simulink model "SWC_FDC_type"  (R2021b)
settings: Solver=FixedStepDiscrete  StartTime=0.0  StopTime=10.0  FixedStep=0.001  RelTol=1e-3
values from neighbouring files (symbols this model uses):
  DID_VCUKey = uint16(0x0202)    [vcu_local_hdr.m]
  DID_XWD = uint16(513)    [vcu_local_hdr.m]
  DIDLen_DKCKey = uint16(8)    [vcu_local_hdr.m]
  DIDLen_DynoMode = uint16(1)    [vcu_local_hdr.m]
  DIDLen_LFLowPresThre = uint16(1)    [vcu_local_hdr.m]
  DIDLen_LFSensorID = uint16(4)    [vcu_local_hdr.m]
  DIDLen_LRLowPresThre = uint16(1)    [vcu_local_hdr.m]
  DIDLen_LRSensorID = uint16(4)    [vcu_local_hdr.m]
  DIDLen_RFLowPresThre = uint16(1)    [vcu_local_hdr.m]
  DIDLen_RFSensorID = uint16(4)    [vcu_local_hdr.m]
  DIDLen_RRLowPresThre = uint16(1)    [vcu_local_hdr.m]
  DIDLen_RRSensorID = uint16(4)    [vcu_local_hdr.m]
  DIDLen_SensorMode = uint16(1)    [vcu_local_hdr.m]
  DIDLen_TPMSLearnSta = uint16(1)    [vcu_local_hdr.m]
  DIDLen_WhlPres = uint16(4)    [vcu_local_hdr.m]
  DIDLen_WhlSensorBattSta = uint16(1)    [vcu_local_hdr.m]
  DIDLen_WhlTmp = uint16(4)    [vcu_local_hdr.m]
  DIDLen_XWDMode = uint16(1)    [vcu_local_hdr.m]
  DIDNum_DKCKey = uint16(0x0202)    [vcu_local_hdr.m]
  DIDNum_DynoMode = uint16(0x0203)    [vcu_local_hdr.m]
  DIDNum_LFLowPresThre = uint16(0x0B08)    [vcu_local_hdr.m]
  DIDNum_LFSensorID = uint16(0x0B01)    [vcu_local_hdr.m]
  DIDNum_LRLowPresThre = uint16(0x0B0A)    [vcu_local_hdr.m]
  DIDNum_LRSensorID = uint16(0x0B03)    [vcu_local_hdr.m]
  DIDNum_RFLowPresThre = uint16(0x0B09)    [vcu_local_hdr.m]
  DIDNum_RFSensorID = uint16(0x0B02)    [vcu_local_hdr.m]
  DIDNum_RRLowPresThre = uint16(0x0B0B)    [vcu_local_hdr.m]
  DIDNum_RRSensorID = uint16(0x0B04)    [vcu_local_hdr.m]
  DIDNum_SensorMode = uint16(0x0B0C)    [vcu_local_hdr.m]
  DIDNum_TPMSLearnSta = uint16(0x0B0D)    [vcu_local_hdr.m]
  DIDNum_WhlPres = uint16(0x0B05)    [vcu_local_hdr.m]
  DIDNum_WhlSensorBattSta = uint16(0x0B07)    [vcu_local_hdr.m]
  DIDNum_WhlTmp = uint16(0x0B06)    [vcu_local_hdr.m]
  DIDNum_XWDMode = uint16(0x0201)    [vcu_local_hdr.m]
  DIDVCUKeyLength = uint16(8)    [vcu_local_hdr.m]
  ENUM_DRIVETRAIN_AWD = uint8(  2  )    [vcu_local_hdr.m]
  ENUM_DRIVETRAIN_FWD = uint8(  1  )    [vcu_local_hdr.m]
  ENUM_DRIVETRAIN_RWD = uint8(  0  )    [vcu_local_hdr.m]
  ENUM_TPMSLearnStatus_LEARNED = uint8(  1  )    [vcu_local_hdr.m]
  ENUM_TPMSLearnStatus_LEARNFAIL = uint8(  2  )    [vcu_local_hdr.m]
  ENUM_TPMSLearnStatus_NOTLEARN = uint8(  0  )    [vcu_local_hdr.m]
  ENUM_TPMSSTA_FAT = uint8(  8  )    [vcu_local_hdr.m]
  ENUM_TPMSSTA_LOWBATTERY = uint8(  2  )    [vcu_local_hdr.m]
  FALSE = boolean( 0 )    [vcu_local_hdr.m]
  ONE_INT = uint8(1)    [vcu_local_hdr.m]
  P_boolean = 0.0    [APPTypes.sldd]
  TRUE = boolean( 1 )    [vcu_local_hdr.m]
  ZERO_FLOAT = single(0)    [vcu_local_hdr.m]
  ZERO_INT = uint8(0)    [vcu_local_hdr.m]
undefined symbols (not defined in the file or in its folder): f32_ApsOutVehSpdSig, KHAL_DKCDecryptEnable_flg_ovrdflg, KHAL_DKCDecryptEnable_flg_ovrdval, KHAL_RandomNumberY1_enum, KHAL_RandomNumberY2_enum, KHAL_RandomNumberY_ovrdflg, KHAL_TPMSRESBUTT_flg_ovrdflg, KHAL_TPMSRESBUTT_flg_ovrdval, R_DIDWriteCDD_CSOP_DIDSet_DKCKey, R_DIDWriteCDD_CSOP_DIDSet_DynoMode, R_DIDWriteCDD_CSOP_DIDSet_LFLowPresThre, R_DIDWriteCDD_CSOP_DIDSet_LFSensorID, R_DIDWriteCDD_CSOP_DIDSet_LRLowPresThre, R_DIDWriteCDD_CSOP_DIDSet_LRSensorID, R_DIDWriteCDD_CSOP_DIDSet_RFLowPresThre, R_DIDWriteCDD_CSOP_DIDSet_RFSensorID, R_DIDWriteCDD_CSOP_DIDSet_RRLowPresThre, R_DIDWriteCDD_CSOP_DIDSet_RRSensorID, R_DIDWriteCDD_CSOP_DIDSet_SensorMode, R_DIDWriteCDD_CSOP_DIDSet_TPMSLearnSta, R_DIDWriteCDD_CSOP_DIDSet_WhlPres, R_DIDWriteCDD_CSOP_DIDSet_WhlSensorBattSta, R_DIDWriteCDD_CSOP_DIDSet_WhlTmp, R_DIDWriteCDD_CSOP_DIDSet_XWDMode, R_E2E_CAN3_VCU1_CSOP_Write_CAN3_VCU1, R_E2E_CAN4_VCU1_CSOP_Write_CAN4_VCU1, R_FDCCDD_Inner_CSOP_FDC_AppCallSleep, R_HALIN_IMU_CSOP_IMUSetSta, R_HALINCDD_CSOP_PAS_Handler, R_HALINCDD_CSOP_UDS_Main, R_HALOUT_APS_CSOP_ApsOutput, R_HALOUTCDD_CSOP_AppNmStateReq, R_HALOUTCDD_CSOP_IVIReset, R_HALOUTCDD_CSOP_SetAcoreRebootCmdACK, R_HALOUTCDD_CSOP_SetSysPwrStat, R_HALOUTCDD_CSOP_SleepRequest, R_NVMReadCDD_Inner_NVM_ReadOperation, R_NVMWriteCDD_Inner_NVM_WriteOperation, R_UDSCDD_CSOP_DdmRestartOperationCycle, R_WDGCDD_CSOP_Call_Watchdog, R_WDGCDD_CSOP_Call_WDG_AppEnd, R_WDGCDD_CSOP_Call_WDG_AppStart, u16_DIDLen_DKCKey, u16_DIDLen_DynoMode, u16_DIDLen_LFLowPresThre, u16_DIDLen_LFSensorID, u16_DIDLen_LRLowPresThre, u16_DIDLen_LRSensorID, u16_DIDLen_RFLowPresThre, u16_DIDLen_RFSensorID, u16_DIDLen_RRLowPresThre, u16_DIDLen_RRSensorID, u16_DIDLen_SensorMode, u16_DIDLen_TPMSLearnSta, u16_DIDLen_WhlPres, u16_DIDLen_WhlSensorBattSta, u16_DIDLen_WhlTmp, u16_DIDLen_XWDMode, u16_DIDNum_DKCKey, u16_DIDNum_DynoMode ... (+42)
libraries: simulink x215, FVT_lib x137, hcu_lib x12, hdlsllib x9, app x1, halin x1, halout x1, inp x1, outp x1
(part 6 of 11)

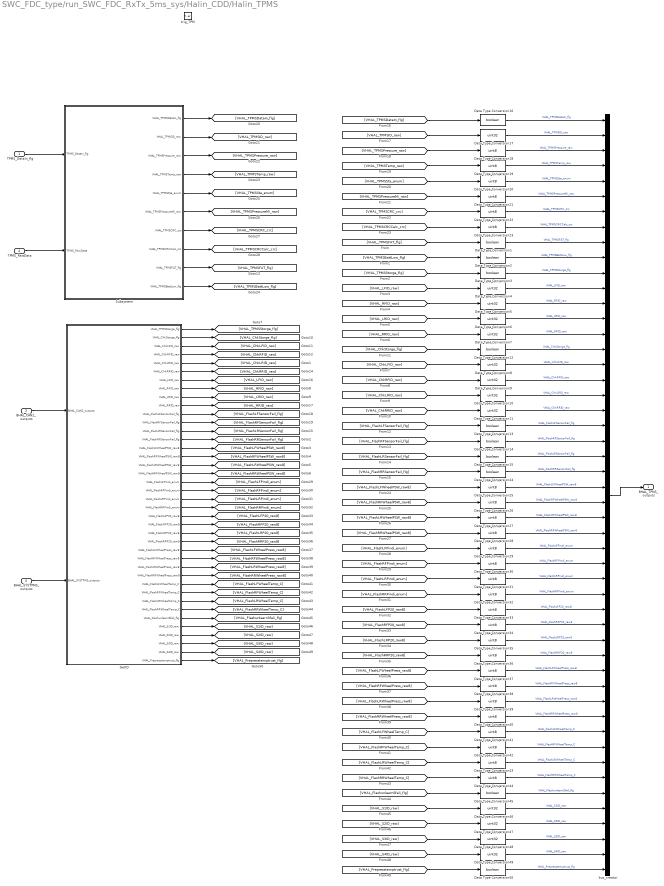
== system SWC_FDC_type/run_SWC_FDC_RxTx_5ms_sys/Halin_CDD/Halin_TPMS ==
  TPMS_DataIn_flg : Inport
  TPMS_RawData : Inport  Port=2
  BHAL_CAN2_outputs : Inport  Port=3
  BHAL_SYSTPMS_outputs : Inport  Port=4
  trig_TPM : TriggerPort  TriggerType=function-call  VariantControl=(inherit)
  Data Type Conversion{1..3,12..16,24,45,50} (11 alike) : DataTypeConversion  OutDataTypeStr=boolean
  Data Type Conversion{4..11,17,46..49} (13 alike) : DataTypeConversion  OutDataTypeStr=uint32
  Data Type Conversion{18..23,25..44} (26 alike) : DataTypeConversion  OutDataTypeStr=uint8
  GetID : Subsystem
  Subsystem : Subsystem
  bus_creator : BusCreator  Inputs=50  OutDataTypeStr=Bus: BHAL_TPMS_outputs  NonVirtualBus=on
  BHAL_TPMS_outputs : Outport
  wires:
  Subsystem/8(VHAL_TPMSCRCCalc_crc) -> [VHAL_TPMSCRCCalc_crc]
  Subsystem/7(VHAL_TPMSCRC_crc) -> [VHAL_TPMSCRC_crc]
  Subsystem/1(VHAL_TPMSDataIn_flg) -> [VHAL_TPMSDataIn_flg]
  Subsystem/9(VHAL_TPMSFAT_flg) -> [VHAL_TPMSFAT_flg]
  Subsystem/2(VHAL_TPMSID_raw) -> [VHAL_TPMSID_raw]
  Subsystem/10(VHAL_TPMSBattLow_flg) -> [VHAL_TPMSBattLow_flg]
  Subsystem/4(VHAL_TPMSTemp_raw) -> [VHAL_TPMSTemp_raw]
  Subsystem/5(VHAL_TPMSSta_enum) -> [VHAL_TPMSSta_enum]
  Subsystem/3(VHAL_TPMSPressure_raw) -> [VHAL_TPMSPressure_raw]
  Subsystem/6(VHAL_TPMSPressureMi_raw) -> [VHAL_TPMSPressureMi_raw]
  TPMS_DataIn_flg/1 -> Subsystem/1(TPMS_DataIn_flg)
  TPMS_RawData/1 -> Subsystem/2(TPMS_RawData)
  Data Type Conversion29/1 -> bus_creator/29  "VHAL_FlashLFPindi_enum"
  GetID/20(VHAL_FlashRFPindi_enum) -> [VHAL_FlashRFPindi_enum]
  GetID/32(VHAL_FlashRFWheelTemp_C) -> [VHAL_FlashRFWheelTemp_C]
  Data Type Conversion2/1 -> bus_creator/10  "VHAL_TPMSBattLow_flg"
  BHAL_CAN2_outputs/1 -> GetID/1(BHAL_CAN2_outputs)
  [VHAL_TPMSBattLow_flg] -> Data Type Conversion2/1
  [VHAL_FlashLRPindi_enum] -> Data Type Conversion31/1
  [VHAL_FlashunlearnSfali_flg] -> Data Type Conversion45/1
  [VHAL_FlashLFPindi_enum] -> Data Type Conversion29/1
  Data Type Conversion28/1 -> bus_creator/28  "VHAL_FlashRRWheelPSW_raw8"
  [VHAL_FlashLFP20_raw8] -> Data Type Conversion33/1
  [VHAL_RRID_raw] -> Data Type Conversion7/1
  Data Type Conversion42/1 -> bus_creator/42  "VHAL_FlashRFWheelTemp_C"
  Data Type Conversion27/1 -> bus_creator/27  "VHAL_FlashLRWheelPSW_raw8"
  [VHAL_FlashLFWheelTemp_C] -> Data Type Conversion41/1
  Data Type Conversion26/1 -> bus_creator/26  "VHAL_FlashRFWheelPSW_raw8"
  [VHAL_FlashRRP20_raw8] -> Data Type Conversion36/1
  GetID/16(VHAL_FlashRFWheelPSW_raw8) -> [VHAL_FlashRFWheelPSW_raw8]
  [VHAL_RFID_raw] -> Data Type Conversion5/1
  Data Type Conversion33/1 -> bus_creator/33  "VHAL_FlashLFP20_raw8"
  Data Type Conversion24/1 -> bus_creator/24  "VHAL_FlashRRSensorFail_flg"
  Data Type Conversion44/1 -> bus_creator/44  "VHAL_FlashRRWheelTemp_C"
  Data Type Conversion34/1 -> bus_creator/34  "VHAL_FlashRFP20_raw8"
  Data Type Conversion45/1 -> bus_creator/45  "VHAL_FlashunlearnSfali_flg"
  GetID/9(VHAL_LRID_raw) -> [VHAL_LRID_raw]
  Data Type Conversion41/1 -> bus_creator/41  "VHAL_FlashLFWheelTemp_C"
  GetID/15(VHAL_FlashLFWheelPSW_raw8) -> [VHAL_FlashLFWheelPSW_raw8]
  Data Type Conversion15/1 -> bus_creator/23  "VHAL_FlashLRSensorFail_flg"
  [VHAL_FlashLRWheelPress_raw8] -> Data Type Conversion39/1
  Data Type Conversion14/1 -> bus_creator/22  "VHAL_FlashRFSensorFail_flg"
  GetID/34(VHAL_FlashRRWheelTemp_C) -> [VHAL_FlashRRWheelTemp_C]
  Data Type Conversion13/1 -> bus_creator/21  "VHAL_FlashLFSensorFail_flg"
  Data Type Conversion32/1 -> bus_creator/32  "VHAL_FlashRRPindi_enum"
  Data Type Conversion31/1 -> bus_creator/31  "VHAL_FlashLRPindi_enum"
  Data Type Conversion16/1 -> bus_creator/1  "VHAL_TPMSDataIn_flg"
  GetID/22(VHAL_FlashRRPindi_enum) -> [VHAL_FlashRRPindi_enum]
  [VHAL_FlashRFSensorFail_flg] -> Data Type Conversion14/1
  GetID/18(VHAL_FlashRRWheelPSW_raw8) -> [VHAL_FlashRRWheelPSW_raw8]
  Data Type Conversion43/1 -> bus_creator/43  "VHAL_FlashLRWheelTemp_C"
  Data Type Conversion22/1 -> bus_creator/7  "VHAL_TPMSCRC_crc"
  Data Type Conversion40/1 -> bus_creator/40  "VHAL_FlashRRWheelPress_raw8"
  Data Type Conversion39/1 -> bus_creator/39  "VHAL_FlashLRWheelPress_raw8"
  [VHAL_FlashRRPindi_enum] -> Data Type Conversion32/1
  Data Type Conversion38/1 -> bus_creator/38  "VHAL_FlashRFWheelPress_raw8"
  [VHAL_FlashLRP20_raw8] -> Data Type Conversion35/1
  Data Type Conversion35/1 -> bus_creator/35  "VHAL_FlashLRP20_raw8"
  GetID/14(VHAL_FlashRRSensorFail_flg) -> [VHAL_FlashRRSensorFail_flg]
  Data Type Conversion37/1 -> bus_creator/37  "VHAL_FlashLFWheelPress_raw8"
  Data Type Conversion36/1 -> bus_creator/36  "VHAL_FlashRRP20_raw8"
  [VHAL_FlashRRWheelTemp_C] -> Data Type Conversion44/1
  [VHAL_FlashLFWheelPress_raw8] -> Data Type Conversion37/1
  GetID/33(VHAL_FlashLRWheelTemp_C) -> [VHAL_FlashLRWheelTemp_C]
  GetID/26(VHAL_FlashRRP20_raw8) -> [VHAL_FlashRRP20_raw8]
  [VHAL_TPMSFAT_flg] -> Data Type Conversion1/1
  [VHAL_TPMSSta_enum] -> Data Type Conversion20/1
  GetID/25(VHAL_FlashLRP20_raw8) -> [VHAL_FlashLRP20_raw8]
  [VHAL_FlashRRWheelPress_raw8] -> Data Type Conversion40/1
  [VHAL_FlashRFP20_raw8] -> Data Type Conversion34/1
  [VHAL_LFID_raw] -> Data Type Conversion4/1
  [VHAL_FlashRFWheelPSW_raw8] -> Data Type Conversion26/1
  [VHAL_FlashRFWheelTemp_C] -> Data Type Conversion42/1
  [VHAL_FlashLRWheelTemp_C] -> Data Type Conversion43/1
  [VHAL_TPMSCRCCalc_crc] -> Data Type Conversion23/1
  GetID/31(VHAL_FlashLFWheelTemp_C) -> [VHAL_FlashLFWheelTemp_C]
  [VHAL_FlashRRSensorFail_flg] -> Data Type Conversion24/1
  [VHAL_FlashLFSensorFail_flg] -> Data Type Conversion13/1
  GetID/30(VHAL_FlashRRWheelPress_raw8) -> [VHAL_FlashRRWheelPress_raw8]
  Data Type Conversion3/1 -> bus_creator/11  "VHAL_TPMSStorge_flg"
  GetID/29(VHAL_FlashLRWheelPress_raw8) -> [VHAL_FlashLRWheelPress_raw8]
  GetID/21(VHAL_FlashLRPindi_enum) -> [VHAL_FlashLRPindi_enum]
  GetID/1(VHAL_TPMSStorge_flg) -> [VHAL_TPMSStorge_flg]
  [VHAL_FlashRFPindi_enum] -> Data Type Conversion30/1
  GetID/19(VHAL_FlashLFPindi_enum) -> [VHAL_FlashLFPindi_enum]
  GetID/23(VHAL_FlashLFP20_raw8) -> [VHAL_FlashLFP20_raw8]
  Data Type Conversion6/1 -> bus_creator/14  "VHAL_LRID_raw"
  GetID/6(VHAL_ChkRRID_raw) -> [VHAL_ChkRRID_raw]
  [VHAL_TPMSDataIn_flg] -> Data Type Conversion16/1
  GetID/17(VHAL_FlashLRWheelPSW_raw8) -> [VHAL_FlashLRWheelPSW_raw8]
  [VHAL_FlashRFWheelPress_raw8] -> Data Type Conversion38/1
  Data Type Conversion1/1 -> bus_creator/9  "VHAL_TPMSFAT_flg"
  GetID/3(VHAL_ChkLFID_raw) -> [VHAL_ChkLFID_raw]
  GetID/35(VHAL_FlashunlearnSfali_flg) -> [VHAL_FlashunlearnSfali_flg]
  [VHAL_FlashLFWheelPSW_raw8] -> Data Type Conversion25/1
  GetID/8(VHAL_RFID_raw) -> [VHAL_RFID_raw]
  GetID/10(VHAL_RRID_raw) -> [VHAL_RRID_raw]
  Data Type Conversion12/1 -> bus_creator/16  "VHAL_ChkStorge_flg"
  [VHAL_FlashLRWheelPSW_raw8] -> Data Type Conversion27/1
  GetID/7(VHAL_LFID_raw) -> [VHAL_LFID_raw]
  Data Type Conversion18/1 -> bus_creator/3  "VHAL_TPMSPressure_raw"
  Data Type Conversion9/1 -> bus_creator/18  "VHAL_ChkRFID_raw"
  Data Type Conversion10/1 -> bus_creator/19  "VHAL_ChkLRID_raw"
  GetID/11(VHAL_FlashLFSensorFail_flg) -> [VHAL_FlashLFSensorFail_flg]
  GetID/27(VHAL_FlashLFWheelPress_raw8) -> [VHAL_FlashLFWheelPress_raw8]
  Data Type Conversion11/1 -> bus_creator/20  "VHAL_ChkRRID_raw"
  Data Type Conversion7/1 -> bus_creator/15  "VHAL_RRID_raw"
  GetID/4(VHAL_ChkRFID_raw) -> [VHAL_ChkRFID_raw]
  [VHAL_TPMSID_raw] -> Data Type Conversion17/1
  [VHAL_ChkStorge_flg] -> Data Type Conversion12/1
  GetID/28(VHAL_FlashRFWheelPress_raw8) -> [VHAL_FlashRFWheelPress_raw8]
  Data Type Conversion8/1 -> bus_creator/17  "VHAL_ChkLFID_raw"
  [VHAL_ChkRRID_raw] -> Data Type Conversion11/1
  Data Type Conversion4/1 -> bus_creator/12  "VHAL_LFID_raw"
  [VHAL_ChkLRID_raw] -> Data Type Conversion10/1
  [VHAL_ChkLFID_raw] -> Data Type Conversion8/1
  [VHAL_ChkRFID_raw] -> Data Type Conversion9/1
  Data Type Conversion5/1 -> bus_creator/13  "VHAL_RFID_raw"
  [VHAL_LRID_raw] -> Data Type Conversion6/1
  [VHAL_TPMSStorge_flg] -> Data Type Conversion3/1
  GetID/2(VHAL_ChkStorge_flg) -> [VHAL_ChkStorge_flg]
  [VHAL_TPMSCRC_crc] -> Data Type Conversion22/1
  Data Type Conversion19/1 -> bus_creator/4  "VHAL_TPMSTemp_raw"
  BHAL_SYSTPMS_outputs/1 -> GetID/2(BHAL_SYSTPMS_outputs)
  [VHAL_FlashLRSensorFail_flg] -> Data Type Conversion15/1
  Data Type Conversion17/1 -> bus_creator/2  "VHAL_TPMSID_raw"
  Data Type Conversion23/1 -> bus_creator/8  "VHAL_TPMSCRCCalc_crc"
  Data Type Conversion30/1 -> bus_creator/30  "VHAL_FlashRFPindi_enum"
  Data Type Conversion21/1 -> bus_creator/6  "VHAL_TPMSPressureMi_raw"
  GetID/5(VHAL_ChkLRID_raw) -> [VHAL_ChkLRID_raw]
  [VHAL_TPMSTemp_raw] -> Data Type Conversion19/1
  GetID/13(VHAL_FlashLRSensorFail_flg) -> [VHAL_FlashLRSensorFail_flg]
  [VHAL_TPMSPressure_raw] -> Data Type Conversion18/1
  GetID/24(VHAL_FlashRFP20_raw8) -> [VHAL_FlashRFP20_raw8]
  bus_creator/1 -> BHAL_TPMS_outputs/1
  Data Type Conversion20/1 -> bus_creator/5  "VHAL_TPMSSta_enum"
  Data Type Conversion25/1 -> bus_creator/25  "VHAL_FlashLFWheelPSW_raw8"
  [VHAL_TPMSPressureMi_raw] -> Data Type Conversion21/1
  GetID/12(VHAL_FlashRFSensorFail_flg) -> [VHAL_FlashRFSensorFail_flg]
  [VHAL_FlashRRWheelPSW_raw8] -> Data Type Conversion28/1
  GetID/36(VHAL_S1ID_raw) -> [VHAL_S1ID_raw]
  GetID/37(VHAL_S2ID_raw) -> [VHAL_S2ID_raw]
  GetID/38(VHAL_S3ID_raw) -> [VHAL_S3ID_raw]
  GetID/39(VHAL_S4ID_raw) -> [VHAL_S4ID_raw]
  Data Type Conversion46/1 -> bus_creator/46  "VHAL_S1ID_raw"
  Data Type Conversion49/1 -> bus_creator/49  "VHAL_S4ID_raw"
  Data Type Conversion48/1 -> bus_creator/48  "VHAL_S3ID_raw"
  Data Type Conversion47/1 -> bus_creator/47  "VHAL_S2ID_raw"
  [VHAL_S1ID_raw] -> Data Type Conversion46/1
  [VHAL_S2ID_raw] -> Data Type Conversion47/1
  [VHAL_S3ID_raw] -> Data Type Conversion48/1
  [VHAL_S4ID_raw] -> Data Type Conversion49/1
  GetID/40(VHAL_Prepresstemptrust_flg) -> [VHAL_Prepresstemptrust_flg]
  [VHAL_Prepresstemptrust_flg] -> Data Type Conversion50/1
  Data Type Conversion50/1 -> bus_creator/50  "VHAL_Prepresstemptrust_flg"

== system SWC_FDC_type/run_SWC_FDC_RxTx_5ms_sys/Halin_CDD/Subsystem ==
  VHAL_ClearDTCcmd_flg : Inport
  Bus Creator : BusCreator  Inputs=1
  Data Type Conversion : DataTypeConversion  OutDataTypeStr=boolean
  BHAL_DDM_outputs : Outport  OutDataTypeStr=Bus: BHAL_DDM_outputs
  wires:
  VHAL_ClearDTCcmd_flg/1 -> Data Type Conversion/1
  Bus Creator/1 -> BHAL_DDM_outputs/1
  Data Type Conversion/1 -> Bus Creator/1  "VHAL_ClearDTCcmd_flg"

== system SWC_FDC_type/run_SWC_FDC_RxTx_5ms_sys/OUTP_AFTER/APM ==
  BOUTP_outputs : Inport  OutDataTypeStr=Bus: BOUTP_outputs
  Bus Selector : BusSelector  OutputSignals=VOUTP_VehSpeed_kph,VOUTP_ShiftGearPosn_enum,VOUTP_FSOffSw_enum,VOUTP_VehSpeedTimeOut_flg,VOUTP_FSOffSwTimeOut_flg,VOUTP_ChrgPlugSta_enum
  Data Type Conversion : DataTypeConversion  OutDataTypeStr=single
  Data Type Conversion{1..5} (5 alike) : DataTypeConversion  OutDataTypeStr=uint8
  ApsOut_GearPosnSig : Outport
  ApsOut_SendChrgPlugStaSig : Outport  Port=2
  ApsOut_SetFrSensorOnCmd : Outport  Port=3
  ApsOut_SetFrSensorSwTOCmd : Outport  Port=4
  ApsOut_SetVehSpdTOCmd : Outport  Port=5
  ApsOut_VehSpdSig : Outport  Port=6
  wires:
  BOUTP_outputs/1 -> [BOUTP_outputs]
  [BOUTP_outputs] -> Bus Selector/1
  Bus Selector/1 -> Data Type Conversion/1  "<VOUTP_VehSpeed_kph>"
  Bus Selector/2 -> Data Type Conversion1/1  "<VOUTP_ShiftGearPosn_enum>"
  Bus Selector/3 -> Data Type Conversion2/1  "<VOUTP_FSOffSw_enum>"
  Bus Selector/4 -> Data Type Conversion3/1  "<VOUTP_VehSpeedTimeOut_flg>"
  Bus Selector/5 -> Data Type Conversion4/1  "<VOUTP_FSOffSwTimeOut_flg>"
  Data Type Conversion1/1 -> ApsOut_GearPosnSig/1
  Data Type Conversion2/1 -> ApsOut_SetFrSensorOnCmd/1
  Data Type Conversion4/1 -> ApsOut_SetFrSensorSwTOCmd/1
  Data Type Conversion5/1 -> ApsOut_SendChrgPlugStaSig/1
  Bus Selector/6 -> Data Type Conversion5/1  "<VOUTP_ChrgPlugSta_enum>"
  Data Type Conversion/1 -> ApsOut_VehSpdSig/1
  Data Type Conversion3/1 -> ApsOut_SetVehSpdTOCmd/1

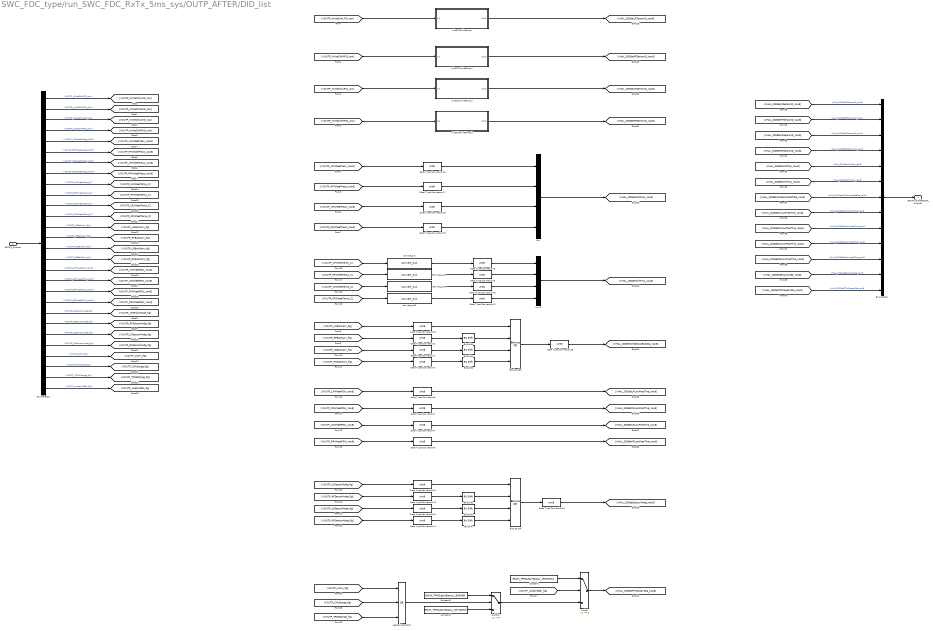
== system SWC_FDC_type/run_SWC_FDC_RxTx_5ms_sys/OUTP_AFTER/DID_list ==
  BOUTP_outputs : Inport
  Bit Shift : hdlsllib/Logic and Bit Operations/Bit Shift  mode=Shift Left Logical  N=3
  Bit Shift1 : hdlsllib/Logic and Bit Operations/Bit Shift  mode=Shift Left Logical  N=2
  Bit Shift2 : hdlsllib/Logic and Bit Operations/Bit Shift  mode=Shift Left Logical  N=1
  Bit Shift3 : hdlsllib/Logic and Bit Operations/Bit Shift  mode=Shift Left Logical  N=3
  Bit Shift4 : hdlsllib/Logic and Bit Operations/Bit Shift  mode=Shift Left Logical  N=2
  Bit Shift5 : hdlsllib/Logic and Bit Operations/Bit Shift  mode=Shift Left Logical  N=1
  Bitwise OR : simulink/Logic and Bit Operations/Bitwise Operator  logicop=OR  UseBitMask=off  NumInputPorts=4  BitMask=bin2dec('11011001')  BitMaskRealWorld=Stored Integer
  Bitwise OR1 : simulink/Logic and Bit Operations/Bitwise Operator  logicop=OR  UseBitMask=off  NumInputPorts=4  BitMask=bin2dec('11011001')  BitMaskRealWorld=Stored Integer
  Bus Creator : BusCreator  Inputs=13
  Bus Selector : BusSelector  OutputSignals=VOUTP_WriteChkLFID_raw,VOUTP_WriteChkRFID_raw,VOUTP_WriteChkLRID_raw,VOUTP_WriteChkRRID_raw,VOUTP_LFWheelPress_raw8,VOUTP_RFWheelPress_raw8,VOUTP_LRWheelPress_raw8,VOUTP_RRWheelPress_raw8,VOUTP_LFWheelTemp_C,VOUTP_RFWheelTemp_C,VOUTP_LRWheelTemp_C,VOUTP_RRWheelTemp_C,VOUTP_LFBatWarn_flg,VOUTP_RFBatWarn_flg,VOUTP_LRBatWarn_flg,VOUTP_RRBatWarn_flg,VOUTP_LFWheelPSW_raw8,VOUTP_LRWheelPSW_raw8,VOUTP_RFWheelPSW_raw8,VOUTP_RRWheelPSW_raw8,VOUTP_LFSensorMode_flg,VOUTP_RFSensorMode_flg,VOUTP_LRSensorMode_flg,VOUTP_RRSensorMode_flg,VOUTP_ALFin_flg,VOUTP_ChkStorge_flg,VOUTP_TPMSStorge_flg,VOUTP_unlearnSfali_flg
  Constant : Constant  Value=ENUM_TPMSLearnStatus_LEARNFAIL
  Constant1 : Constant  Value=ENUM_TPMSLearnStatus_NOTLEARN
  Constant2 : Constant  Value=ENUM_TPMSLearnStatus_LEARNED
  Data Type Conversion{1..22} (22 alike) : DataTypeConversion  OutDataTypeStr=uint8
  Logical Operator1 : Logic  Operator=OR  Inputs=3  AllPortsSameDT=off  OutDataTypeStr=boolean
  Mux : Mux
  Mux2 : Mux
  Switch : Switch  Criteria=u2 ~= 0
  Switch1 : Switch  Criteria=u2 ~= 0
  convert_out{,1..3} (4 alike) : FVT_lib/hal/convert_out  gain=1  offset=-40
  uint32Touint8Array : Subsystem
  uint32Touint8Array1 : Subsystem
  uint32Touint8Array2 : Subsystem
  uint32Touint8Array3 : Subsystem
  BOUTP_DIDSetData_outputs : Outport
  wires:
  BOUTP_outputs/1 -> Bus Selector/1
  Bus Selector/1 -> [VOUTP_WriteChkLFID_raw]  "<VOUTP_WriteChkLFID_raw>"
  Bus Selector/2 -> [VOUTP_WriteChkRFID_raw]  "<VOUTP_WriteChkRFID_raw>"
  Bus Selector/4 -> [VOUTP_WriteChkRRID_raw]  "<VOUTP_WriteChkRRID_raw>"
  Bus Selector/3 -> [VOUTP_WriteChkLRID_raw]  "<VOUTP_WriteChkLRID_raw>"
  Bus Selector/5 -> [VOUTP_LFWheelPress_raw8]  "<VOUTP_LFWheelPress_raw8>"
  Bus Selector/6 -> [VOUTP_RFWheelPress_raw8]  "<VOUTP_RFWheelPress_raw8>"
  Bus Selector/7 -> [VOUTP_LRWheelPress_raw8]  "<VOUTP_LRWheelPress_raw8>"
  Bus Selector/8 -> [VOUTP_RRWheelPress_raw8]  "<VOUTP_RRWheelPress_raw8>"
  Bus Selector/13 -> [VOUTP_LFBatWarn_flg]  "<VOUTP_LFBatWarn_flg>"
  Bus Selector/14 -> [VOUTP_RFBatWarn_flg]  "<VOUTP_RFBatWarn_flg>"
  Bus Selector/15 -> [VOUTP_LRBatWarn_flg]  "<VOUTP_LRBatWarn_flg>"
  Bus Selector/16 -> [VOUTP_RRBatWarn_flg]  "<VOUTP_RRBatWarn_flg>"
  Bus Selector/18 -> [VOUTP_LRWheelPSW_raw8]  "<VOUTP_LRWheelPSW_raw8>"
  Bus Selector/19 -> [VOUTP_RFWheelPSW_raw8]  "<VOUTP_RFWheelPSW_raw8>"
  Bus Selector/20 -> [VOUTP_RRWheelPSW_raw8]  "<VOUTP_RRWheelPSW_raw8>"
  Bus Selector/17 -> [VOUTP_LFWheelPSW_raw8]  "<VOUTP_LFWheelPSW_raw8>"
  Bus Selector/21 -> [VOUTP_LFSensorMode_flg]  "<VOUTP_LFSensorMode_flg>"
  Bus Selector/22 -> [VOUTP_RFSensorMode_flg]  "<VOUTP_RFSensorMode_flg>"
  Bus Selector/23 -> [VOUTP_LRSensorMode_flg]  "<VOUTP_LRSensorMode_flg>"
  Bus Selector/24 -> [VOUTP_RRSensorMode_flg]  "<VOUTP_RRSensorMode_flg>"
  Bus Selector/27 -> [VOUTP_TPMSStorge_flg]  "<VOUTP_TPMSStorge_flg>"
  Bus Selector/25 -> [VOUTP_ALFin_flg]  "<VOUTP_ALFin_flg>"
  Bus Selector/26 -> [VOUTP_ChkStorge_flg]  "<VOUTP_ChkStorge_flg>"
  Bus Selector/28 -> [VOUTP_unlearnSfali_flg]  "<VOUTP_unlearnSfali_flg>"
  Bus Selector/9 -> [VOUTP_LFWheelTemp_C]  "<VOUTP_LFWheelTemp_C>"
  Bus Selector/10 -> [VOUTP_RFWheelTemp_C]  "<VOUTP_RFWheelTemp_C>"
  Bus Selector/11 -> [VOUTP_LRWheelTemp_C]  "<VOUTP_LRWheelTemp_C>"
  Bus Selector/12 -> [VOUTP_RRWheelTemp_C]  "<VOUTP_RRWheelTemp_C>"
  Data Type Conversion8/1 -> Mux2/1
  Data Type Conversion9/1 -> Mux2/2
  Data Type Conversion10/1 -> Mux2/3
  Data Type Conversion11/1 -> Mux2/4
  [VOUTP_LFWheelPSW_raw8] -> Data Type Conversion6/1
  [VOUTP_RRWheelPSW_raw8] -> Data Type Conversion5/1
  [VOUTP_LFSensorMode_flg] -> Data Type Conversion21/1
  [VOUTP_RRSensorMode_flg] -> Data Type Conversion14/1
  [VOUTP_LRSensorMode_flg] -> Data Type Conversion12/1
  [VOUTP_RFSensorMode_flg] -> Data Type Conversion13/1
  Data Type Conversion21/1 -> Bitwise OR/1
  Data Type Conversion12/1 -> Bit Shift1/1
  Data Type Conversion14/1 -> Bit Shift/1
  Constant1/1 -> Switch1/3
  [VOUTP_ALFin_flg] -> Logical Operator1/1
  Switch1/1 -> Switch/3
  [VOUTP_ChkStorge_flg] -> Logical Operator1/2
  Constant/1 -> Switch/1
  Constant2/1 -> Switch1/1
  [VOUTP_TPMSStorge_flg] -> Logical Operator1/3
  Logical Operator1/1 -> Switch1/2
  [VOUTP_unlearnSfali_flg] -> Switch/2
  Mux/1 -> [VHAL_DIDSetWhlPres_raw8]
  Mux2/1 -> [VHAL_DIDSetWhlTmp_raw8]
  Data Type Conversion6/1 -> [VHAL_DIDSetLFLowPresThre_raw8]
  Data Type Conversion7/1 -> [VHAL_DIDSetRFLowPresThre_raw8]
  Data Type Conversion4/1 -> [VHAL_DIDSetLRLowPresThre_raw8]
  Data Type Conversion5/1 -> [VHAL_DIDSetRRLowPresThre_raw8]
  Bitwise OR/1 -> Data Type Conversion20/1
  Switch/1 -> [VHAL_DIDSetTPMSLearnSta_raw8]
  Bit Shift/1 -> Bitwise OR/4
  Bit Shift1/1 -> Bitwise OR/3
  Bit Shift2/1 -> Bitwise OR/2
  Data Type Conversion20/1 -> [VHAL_DIDSetSensorMode_raw8]
  Data Type Conversion13/1 -> Bit Shift2/1
  [VOUTP_RFBatWarn_flg] -> Data Type Conversion2/1
  Data Type Conversion1/1 -> Bit Shift4/1
  [VOUTP_LRBatWarn_flg] -> Data Type Conversion1/1
  [VOUTP_LFBatWarn_flg] -> Data Type Conversion22/1
  Bitwise OR1/1 -> Data Type Conversion15/1
  Bit Shift4/1 -> Bitwise OR1/3
  Data Type Conversion2/1 -> Bit Shift5/1
  Bit Shift3/1 -> Bitwise OR1/4
  Data Type Conversion22/1 -> Bitwise OR1/1
  Data Type Conversion3/1 -> Bit Shift3/1
  Bit Shift5/1 -> Bitwise OR1/2
  [VOUTP_RRBatWarn_flg] -> Data Type Conversion3/1
  Data Type Conversion15/1 -> [VHAL_DIDSetWhlSensorBattSta_raw8]
  [VHAL_DIDSetTPMSLearnSta_raw8] -> Bus Creator/13  "VHAL_DIDSetTPMSLearnSta_raw8"
  [VHAL_DIDSetLFSensorID_raw8] -> Bus Creator/1  "VHAL_DIDSetLFSensorID_raw8"
  [VHAL_DIDSetRFSensorID_raw8] -> Bus Creator/2  "VHAL_DIDSetRFSensorID_raw8"
  [VHAL_DIDSetLRSensorID_raw8] -> Bus Creator/3  "VHAL_DIDSetLRSensorID_raw8"
  [VHAL_DIDSetRRSensorID_raw8] -> Bus Creator/4  "VHAL_DIDSetRRSensorID_raw8"
  [VHAL_DIDSetWhlPres_raw8] -> Bus Creator/5  "VHAL_DIDSetWhlPres_raw8"
  [VHAL_DIDSetWhlTmp_raw8] -> Bus Creator/6  "VHAL_DIDSetWhlTmp_raw8"
  [VHAL_DIDSetWhlSensorBattSta_raw8] -> Bus Creator/7  "VHAL_DIDSetWhlSensorBattSta_raw8"
  [VHAL_DIDSetLFLowPresThre_raw8] -> Bus Creator/8  "VHAL_DIDSetLFLowPresThre_raw8"
  [VHAL_DIDSetRFLowPresThre_raw8] -> Bus Creator/9  "VHAL_DIDSetRFLowPresThre_raw8"
  [VHAL_DIDSetLRLowPresThre_raw8] -> Bus Creator/10  "VHAL_DIDSetLRLowPresThre_raw8"
  [VHAL_DIDSetRRLowPresThre_raw8] -> Bus Creator/11  "VHAL_DIDSetRRLowPresThre_raw8"
  [VHAL_DIDSetSensorMode_raw8] -> Bus Creator/12  "VHAL_DIDSetSensorMode_raw8"
  Bus Creator/1 -> BOUTP_DIDSetData_outputs/1
  [VOUTP_WriteChkLFID_raw] -> uint32Touint8Array/1(In1)
  uint32Touint8Array/1(Out1) -> [VHAL_DIDSetLFSensorID_raw8]
  [VOUTP_WriteChkRFID_raw] -> uint32Touint8Array1/1(In1)
  uint32Touint8Array1/1(Out1) -> [VHAL_DIDSetRFSensorID_raw8]
  [VOUTP_WriteChkLRID_raw] -> uint32Touint8Array2/1(In1)
  uint32Touint8Array2/1(Out1) -> [VHAL_DIDSetLRSensorID_raw8]
  [VOUTP_WriteChkRRID_raw] -> uint32Touint8Array3/1(In1)
  uint32Touint8Array3/1(Out1) -> [VHAL_DIDSetRRSensorID_raw8]
  [VOUTP_RFWheelPress_raw8] -> Data Type Conversion17/1
  [VOUTP_LFWheelPress_raw8] -> Data Type Conversion16/1
  [VOUTP_LRWheelPress_raw8] -> Data Type Conversion18/1
  [VOUTP_RRWheelPress_raw8] -> Data Type Conversion19/1
  convert_out/1 -> Data Type Conversion8/1
  convert_out1/1 -> Data Type Conversion9/1
  convert_out2/1 -> Data Type Conversion10/1
  convert_out3/1 -> Data Type Conversion11/1
  Data Type Conversion16/1 -> Mux/1
  Data Type Conversion17/1 -> Mux/2
  Data Type Conversion18/1 -> Mux/3
  Data Type Conversion19/1 -> Mux/4
  [VOUTP_LFWheelTemp_C] -> convert_out/1
  [VOUTP_RFWheelTemp_C] -> convert_out1/1
  [VOUTP_LRWheelTemp_C] -> convert_out2/1
  [VOUTP_RRWheelTemp_C] -> convert_out3/1
  [VOUTP_RFWheelPSW_raw8] -> Data Type Conversion7/1
  [VOUTP_LRWheelPSW_raw8] -> Data Type Conversion4/1
